simulink model "ramper"  (Simulink 6.6)
settings: Solver=ode3  SolverMode=SingleTasking  StartTime=0.0  StopTime=2  FixedStep=sample  RelTol=1e-3
undefined symbols (not defined in the file or in its folder): sample
settings Model: Creator=Tommy  LastModifiedBy=Tommy

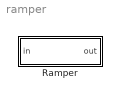
== system ramper ==
  Ramper : Subsystem  mask{ramps=8, samplerate=sample, u_old=[0;0]}
      mask prompts: ramps "Total ramp steps"; samplerate "Sample rate"; u_old "Dimensions"
      mask help:
      | Signal ramper
      |
      | Sample rate should be the sample rate of the system
      | The source signal sample rate should be the sample rate * total ramp steps
      | Set Dimension variable to an empty array of required size, ie. [0;0;0] for 3 dimensions

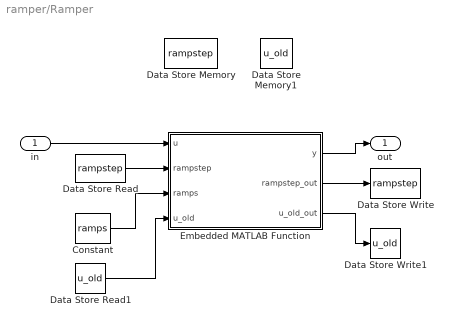
== system ramper/Ramper ==
  in : Inport
  Constant : Constant  Value=ramps  SampleTime=samplerate
  Data Store Memory : DataStoreMemory  DataStoreName=rampstep  InitialValue=1
  Data Store Memory1 : DataStoreMemory  DataStoreName=u_old  InitialValue=u_old
  Data Store Read : DataStoreRead  DataStoreName=rampstep  SampleTime=samplerate
  Data Store Read1 : DataStoreRead  DataStoreName=u_old  SampleTime=samplerate
  Data Store Write : DataStoreWrite  DataStoreName=rampstep  SampleTime=samplerate
  Data Store Write1 : DataStoreWrite  DataStoreName=u_old  SampleTime=samplerate
  Embedded MATLAB Function : Stateflow chart
  out : Outport
  wires:
  in/1 -> Embedded MATLAB Function/1(u)
  Data Store Read/1 -> Embedded MATLAB Function/2(rampstep)
  Constant/1 -> Embedded MATLAB Function/3(ramps)
  Data Store Read1/1 -> Embedded MATLAB Function/4(u_old)
  Embedded MATLAB Function/2(rampstep_out) -> Data Store Write/1
  Embedded MATLAB Function/3(u_old_out) -> Data Store Write1/1
  Embedded MATLAB Function/1(y) -> out/1

== matlab function Ramper/Embedded MATLAB Function ==
  data: u input inherited; y output inherited; rampstep input inherited; ramps input inherited; u_old input inherited; rampstep_out output inherited; u_old_out output inherited
function [y,rampstep_out,u_old_out] = fcn(u,rampstep,ramps,u_old)

%% Ramp
y = (u - u_old)/ramps * rampstep + u_old;    
    
%% Reset ramper
if (rampstep == ramps)
    rampstep_out = 1;
    u_old_out = u; %save this displacement for the base of the next ramped command
else
    rampstep_out = rampstep + 1;
    u_old_out = u_old;
end
